simulink subsystem "OneMotorPower"  (R2021b)
settings: Solver=VariableStepAuto  StartTime=0.0  StopTime=10.0  RelTol=1e-3
settings Model: Creator=tsuyoshi  LastModifiedBy=FEM

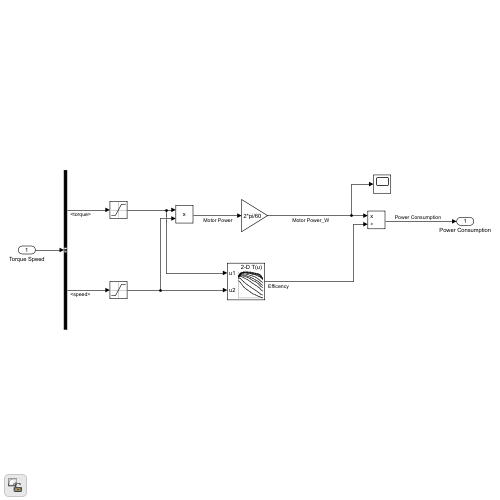
[thumbnail: Simulink's stored preview of the top-level diagram]
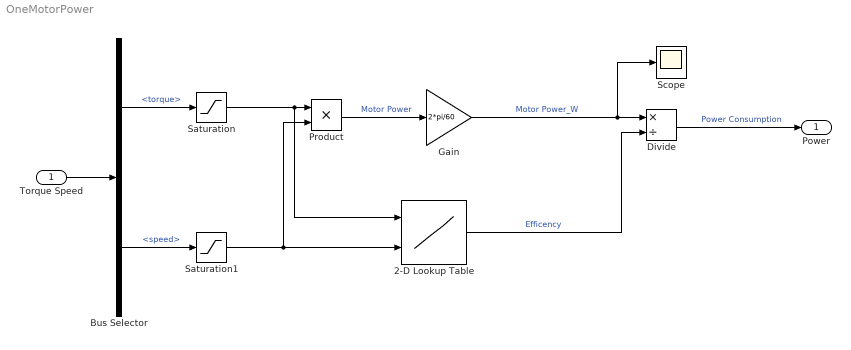
== system OneMotorPower ==
  Torque Speed : Inport
  2-D Lookup Table : Lookup_n-D  BreakpointsForDimension1="[1.3000    2.7000    5.4000    7.9000   10.4000   12.5000   14.4000   16.0000   17.4000   18.5000   19.6000]"  BreakpointsForDimension2="[ 500        1000        2000        3000        4000        6000       10000       12000       15000       19000]"  Table=|  InternalRulePriority=Speed  RndMeth=Simplest  InputSameDT=on
      | [ 0.6437    0.7133    0.7364    0.7470    0.7543    0.7657    0.7700    0.7708    0.7756    0.7814
      |     0.5842    0.7048    0.7757    0.8040    0.8201    0.8392    0.8516    0.8544    0.8597    0.8650
      |     0.4494    0.6081    0.7335    0.7882    0.8194    0.8543    0.8820    0.8888    0.8971    0.9044
      |     0.3559    0.5190    0.6702    0.7426    0.7854    0.8342    0.8758    0.8865    0.8984    0.9086
      |     0.2914    0.4478    0.6101    0.6941    0.7457    0.8062    0.8593    0.8758    0.8886    0.9016
      |     0.2417    0.3871    0.5522    0.6439    0.7024    0.7730    0.8373    0.8548    0.8737    0.8898
      |     0.2041    0.3371    0.5004    0.5965    0.6599    0.7388    0.8133    0.8342    0.8566    0.8759
      |     0.1731    0.2940    0.4510    0.5487    0.6155    0.7010    0.7856    0.8097    0.8356    0.8581
      |     0.1482    0.2575    0.4067    0.5041    0.5728    0.6634    0.7570    0.7840    0.8134    0.8271
      |     0.1281    0.2267    0.3672    0.4630    0.5325    0.6267    0.7277    0.7575    0.7902    0.7696
      |     0.1117    0.2005    0.3321    0.4251    0.4944    0.5909    0.6982    0.7306    0.6766    0.6928]
      settings: InputPortMap=u0,u1
  Bus Selector : BusSelector  OutputSignals=torque,speed
  Divide : Product  Inputs=*/
  Gain : Gain  Gain=2*pi/60
  Product : Product
  Saturation : Saturate  UpperLimit=21  LowerLimit=0
  Saturation1 : Saturate  UpperLimit=19000  LowerLimit=0
  Scope : Scope
  Power : Outport  VectorParamsAs1DForOutWhenUnconnected=off
  wires:
  Gain/1 -> Divide/1, Scope/1  "Motor Power_W"
  Bus Selector/1 -> Saturation/1  "<torque>"
  Bus Selector/2 -> Saturation1/1  "<speed>"
  Divide/1 -> Power/1  "Power Consumption"
  Product/1 -> Gain/1  "Motor Power"
  2-D Lookup Table/1 -> Divide/2  "Efficency"
  Saturation/1 -> Product/1, 2-D Lookup Table/1
  Saturation1/1 -> 2-D Lookup Table/2, Product/2
  Torque Speed/1 -> Bus Selector/1
